simulink model "Main_model"  (R2021b)
settings: Solver=ode23t  StartTime=0.0  StopTime=sim_t_end  RelTol=1e-3
undefined symbols (not defined in the file): ambient_co2, ambient_pressure, ambient_rh, ambient_temp, battery, battery_heat_gen_scale, battery_mass, battery_thermal_mass, cab_air_v_dot, cabin_heater_cmd, cabin_heater_max_power, case_cold_plate_mass, case_cold_plate_thermal_mass, chiller_baffles_n, chiller_tube_length, chiller_tubes_n_rows, compressor_max_m_dot, compressor_ref_m_dot, condenser_air_min_flow_area, condenser_tube_width, const_current, coolant_channel_length, coolant_initial_T, coolant_m_dot, coolant_pipe_cross_sec_area, evaporator_air_cross_sec_area, evaporator_air_min_flow_area, evaporator_tube_width, motor_mc_heat_fraction, n_parallel, power_fraction_rear, ptc_heater_max_power, ptc_heater_thermal_mass, rad_air_v_dot, radiator_air_cross_sec_area, radiator_air_min_flow_area, radiator_tube_width, ref_m_dot, ref_pipe_dia, refrigerant_initial_void_fraction, refrigerant_pipe_cross_sec_area, T_bat_active_cool, T_bat_active_heat, T_bat_passive_cool, T_bat_passive_heat, T_battery_init, T_battery_nom, T_cabin_init, T_cabin_setpoint, T_dcdc_nom, T_DT_high, T_DT_passive_cool, T_DT_whr_active, T_front_gb_nom, T_front_mc_nom, T_front_motor_nom, T_rear_gb_nom, T_rear_mc_nom, T_rear_motor_nom, three_w_valve_max_open_area_factor ... (+3)
libraries: fl_lib x448, nesl_utility x328, SimscapeFluids_lib x134, slpidlib x15, ee_lib x9, simulink x8, LiBatteryElements_lib x4, SignalEditorBlockLib x1
(part 24 of 24)

== matlab function Main_model/HP Control Systems Only DT to Chiller WHR/Valves Control ==
  data: v1 output; v2 output; v3 output; v4 output; v5 output; v6 output; v7 output; v8 output; v9 output; v10 output; T_cabin input; T_amb input; T_battery input; T_DT_max input; T_DT_min input; current_mode output; T_bat_passive_cool parameter; T_DT_whr_active parameter; T_bat_active_cool parameter; T_bat_passive_heat parameter; T_DT_passive_cool parameter; T_DT_high parameter; T_cabin_setpoint parameter
function [v1,v2,v3,v4,v5,v6,v7,v8,v9,v10,current_mode]= fcn(T_cabin, T_amb, T_battery, T_DT_max, T_DT_min, T_bat_passive_cool, T_DT_whr_active, T_bat_active_cool, T_bat_passive_heat, T_DT_passive_cool, T_DT_high,T_cabin_setpoint)

if T_amb<T_cabin_setpoint-273
    if T_battery<T_bat_passive_heat
        if T_DT_min<T_DT_whr_active
            mode(1)
        elseif T_DT_max<T_DT_high
            mode(2)
        else 
            mode(2.25)
        end
    elseif T_battery >=T_bat_passive_heat && T_battery<=T_bat_passive_cool
        if T_DT_min<T_DT_whr_active
            mode(3)
        elseif T_DT_max<T_DT_high
            mode(4)            
        else 
            mode(4.25)
        end
    else
        if T_DT_min<T_DT_whr_active
            mode(5)
        elseif T_DT_max<T_DT_high
            mode(6)            
        else 
            mode(6.25)
        end
    end

elseif T_amb >=17 && T_cabin<=23
    if T_battery<T_bat_passive_cool
        if T_DT_max<=T_DT_passive_cool
            mode(10)
        else
            mode(10.25)
        end
    else
        if T_battery>=T_bat_passive_cool && T_battery<=T_bat_active_cool
            if T_DT_max<=T_DT_passive_cool
                mode(9)
            else
                mode(8)
            end            
        else
            if T_DT_max<=T_DT_passive_cool
                mode(9.25)
            else
                mode(8.25)
            end 
        end
    end

else
    if T_battery<=T_bat_passive_cool
        if T_DT_max<=T_DT_passive_cool
            mode(13)
        else
            mode(13.25)
        end        
    else
        if T_battery>=T_bat_passive_cool && T_battery<=T_bat_active_cool
            if T_DT_max<=T_DT_passive_cool
                mode(12)
            else
                mode(11)
            end            
        else
            if T_DT_max<=T_DT_passive_cool
                mode(12.25)
            else
                mode(11.25)
            end 
        end        
    end

end

    function reset_valves()
        v1=0;
        v2=0;
        v3=0;
        v4=0;
        v5=0;
        v6=0;
        v7=0;
        v8=0;
        v9=0;
        v10=0;
    end
    function mode(x)
        reset_valves()
        if x==1
            v2=1;
            v3=1;
            v6=1;
            current_mode=1;
        elseif x==2
            v3=1;
            v6=1;
            v5=1;
            current_mode=2;          
        elseif x==2.25
            v3=1;
            v6=1;
            v5=1;
            v10=1;
            current_mode=2.25;            
        elseif x==3
            v2=1;
            v3=1;
            current_mode=3;           
        elseif x==4
            v3=1; 
            v5=1;
            current_mode=4;
        elseif x==4.25
            v3=1; 
            v5=1;
            v10=1;
            current_mode=4.25;            
        elseif x==5
            v2=1;
            v3=1;
            v9=1;
            current_mode=5;
        elseif x==6
            v3=1;
            v9=1;
            v5=1;
            current_mode=6;
        elseif x==6.25
            v3=1;
            v9=1;
            v5=1;
            v10=1;
            current_mode=6.25;            
        elseif x==7
            v2=1;
            v6=1;                        
            current_mode=7;
        elseif x==8
            v9=1;
            v10=1;                        
            current_mode=8;
        elseif x==8.25
            v1=1;
            v7=1;              
            v10=1;              
            current_mode=8.25;
        elseif x==9
            v9=1;              
            current_mode=9;
        elseif x==9.25
            v1=1;
            v7=1;              
            current_mode=9.25;
        elseif x==10              
            current_mode=10;
        elseif x==10.25
            v10=1;            
            current_mode=10.25;
        elseif x==11
            v1=1;
            v4=1;
            v9=1;            
            v10=1;            
            current_mode=11;
        elseif x==11.25
            v1=1;
            v4=1;
            v7=1;            
            v10=1;            
            current_mode=11.25;
        elseif x==12
            v1=1;
            v4=1;            
            current_mode=12;
        elseif x==12.25
            v1=1;
            v4=1;
            v7=1;            
            current_mode=12.25;
        elseif x==13
            v1=1;
            v4=1;            
            current_mode=13;
        elseif x==13.25
            v1=1;
            v4=1;           
            v10=1;            
            current_mode=13.25;
        else
            error('Mode not Valid')
        end
    end
end
